simulink model "fm"  (Simulink 10.0)
settings: Solver=ode3  StartTime=0.0  StopTime=10.0  RelTol=1e-3
undefined symbols (not defined in the file): DiscIntNeverNeededParam
libraries: simulink x1
settings Model: Creator=amukh  LastModifiedBy=amukh
settings DataIOCC: SaveFormat=Dataset  ReturnWorkspaceOutputs=on
settings OptimizationCC: LifeSpan=auto
settings DebuggingCC: UnderspecifiedInitializationDetection=Simplified  MergeDetectMultiDrivingBlocksExec=error  SFUnexpectedBacktrackingDiag=error  SFNoUnconditionalDefaultTransitionDiag=error  SFExecutionAtInitializationDiag=warning  ArithmeticOperatorsInVariantConditions=error
settings HardwareCC: ProdBitPerPointer=64  ProdBitPerSizeT=64  ProdBitPerPtrDiffT=64  ProdLargestAtomicFloat=Float  ProdIntDivRoundTo=Zero  ProdEndianess=LittleEndian  ProdWordSize=64  ProdHWDeviceType=Intel->x86-64 (Windows64)
settings ModelReferenceCC: PropagateSignalLabelsOutOfModel=on
settings SFSimCC: SimUseLocalCustomCode=on  CustomCodeUndefinedFunction=FilterOut
settings RTWCC: RTWUseLocalCustomCode=on
settings CodeAppCC: StateflowObjectComments=off
settings GRTTargetCC: TargetLangStandard=C99 (ISO)  CombineOutputUpdateFcns=on  GRTInterface=off
settings ConfigComp: CovMetricSettings=dwe  CovHtmlReporting=off  CovSaveCumulativeToWorkspaceVar=off  CovSaveSingleToWorkspaceVar=off

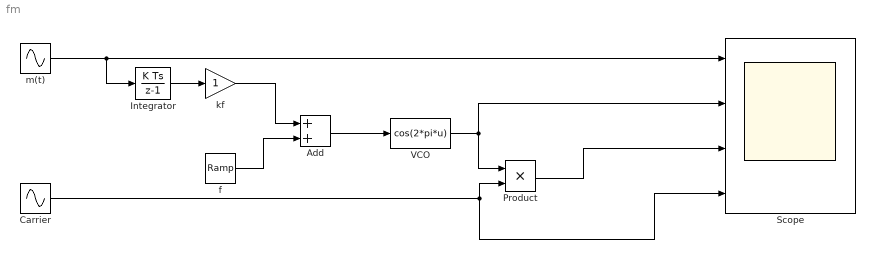
== system fm ==
  "Add " : Sum
  "Carrier " : Sin  Frequency=2.5*2*pi  SampleTime=0
  Integrator : DiscreteIntegrator  SampleTime=0.01  ICPrevOutput=DiscIntNeverNeededParam  ICPrevScaledInput=DiscIntNeverNeededParam
  "Product " : Product
  "Scope " : Scope  NumInputPorts=4
  VCO : Fcn  Expr=cos(2*pi*u)
  f : simulink/Sources/Ramp  slope=10  start=0  InitialOutput=0
  kf : Gain
  m(t) : Sin  Amplitude=20  Frequency=2*pi*20  Phase=pi/2  SampleTime=0
  wires:
  m(t)/1 -> Integrator/1, "Scope "/1
  Integrator/1 -> kf/1
  kf/1 -> "Add "/1
  f/1 -> "Add "/2
  "Add "/1 -> VCO/1
  VCO/1 -> "Product "/1, "Scope "/2
  "Carrier "/1 -> "Scope "/4, "Product "/2
  "Product "/1 -> "Scope "/3
